simulink model "NoPainNoCrane_Software"  (R2016a)
settings: Solver=ode15s  StartTime=0.0  StopTime=80  RelTol=1e-3
values from neighbouring files (symbols this model uses):
  AngleDX = 0    [RunHWModel.m]    (also in simSetup.m; workspace.mat)
  AngleDY = AngleDX    (= 0)    [RunHWModel.m]    (also in simSetup.m; workspace.mat)
  AngleIX = 0    [RunHWModel.m]    (also in simSetup.m; workspace.mat)
  AngleIY = AngleIX    (= 0)    [RunHWModel.m]    (also in simSetup.m; workspace.mat)
  AnglePX = 2.0    (= 2)    [RunHWModel.m]    (also in simSetup.m; workspace.mat)
  AnglePY = AnglePX    (= 2)    [RunHWModel.m]    (also in simSetup.m; workspace.mat)
  DC1x = 0.1    [RunHWModel.m]    (also in simSetup.m; workspace.mat)
  DC1y = DC1x    (= 0.1)    [RunHWModel.m]    (also in simSetup.m; workspace.mat)
  IC1x = 0.9    [RunHWModel.m]    (also in simSetup.m; workspace.mat)
  IC1y = IC1x    (= 0.9)    [RunHWModel.m]    (also in simSetup.m; workspace.mat)
  m = 0.47    [workspace.mat]
  MR = 1.71    [workspace.mat]
  PC1x = 4.7    [RunHWModel.m]    (also in simSetup.m; workspace.mat)
  PC1y = PC1x    (= 4.7)    [RunHWModel.m]    (also in simSetup.m; workspace.mat)
  TxBreak = 0    [setup.m]    (also in workspace.mat)
  TxCoulomb = 2.5    [setup.m]    (also in workspace.mat)
  TxVisc = 49.1750    (= 49.175)    [setup.m]    (also in workspace.mat)
  TyBreak = 0    [setup.m]    (also in workspace.mat)
  TyCoulomb = 1.8    [setup.m]    (also in workspace.mat)
  TzBreak = 0    [workspace.mat]
  TzCoulomb = 6.1    [workspace.mat]
  waypoints = [waypoints is_target]    [path_planning.m]    (also in workspace.mat = [0 0 9 9 10 6 4 8 19 20 20 0 ... (55 elements, 11x5)])
  xRange = [0 0.52]    [workspace.mat]
  xZero = 0    [setup.m]    (also in workspace.mat)
  yRange = [0 0.62]    [workspace.mat]
  yZero = 0    [setup.m]    (also in workspace.mat)
  zRange = [0.17 0.8]    [workspace.mat]
  zZero = 0.47    [workspace.mat]
undefined symbols (not defined in the file or in its folder): X, Y, Z
undefined symbols (not defined in the file): M, TorqueMultX, TorqueMultY, TorqueMultZ, TxTrans, TyTrans, TyVisc, TzTrans, TzVisc
libraries: sm_lib x146, fl_lib x62, nesl_utility x24, simulink x10, elec_lib x9, sm_double_wishbone_suspension_lib x4, aerolibtransform2 x1
(part 1 of 15)
settings Model: Creator=jsustare  LastModifiedBy=Jukka
settings SolverCC: MaxConsecutiveMinStep=10
settings DataIOCC: SaveFormat=StructureWithTime
settings DebuggingCC: AllowSymbolicDim=off
settings ModelReferenceCC: PropagateSignalLabelsOutOfModel=off
settings GRTTargetCC: GeneratePreprocessorConditionals=Use local settings
settings SimscapeCC: SimscapeLogType=all  SimscapeLogLimitData=off
settings ConfigurationSet: Description=SimMechanics 2G

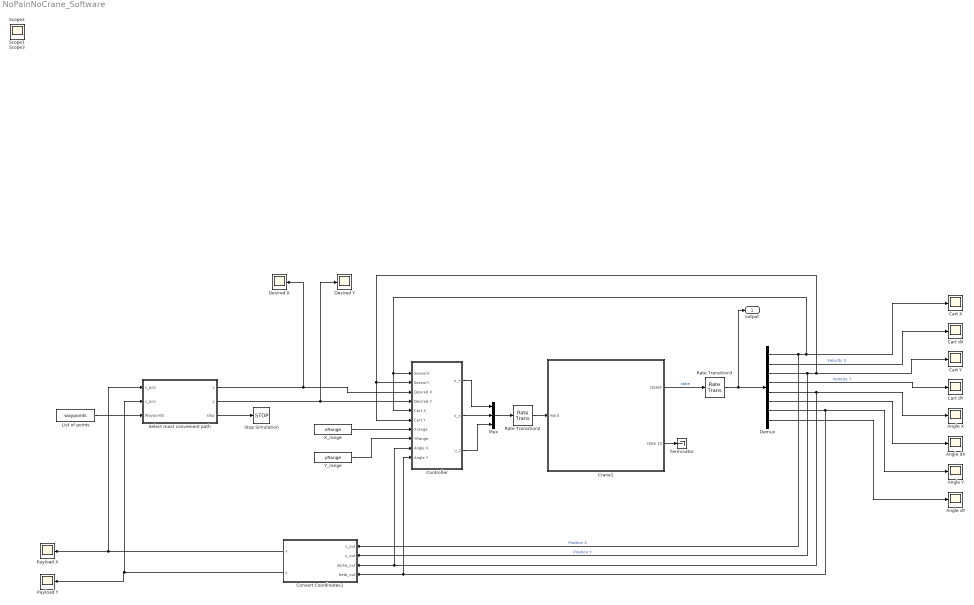
== system NoPainNoCrane_Software ==
  Angle X : Scope
  Angle Y : Scope
  Angle dX : Scope
  Angle dY : Scope
  Cart X : Scope
  Cart Y : Scope
  Cart dX : Scope
  Cart dY : Scope
  Controller : Subsystem
  Convert Coordinates1 : MATLAB Function  TreatAsAtomicUnit=on
  Crane1 : Subsystem  mask{penduMass=m, cartMass=M, MR=MR, xRange=xRange, yRange=yRange, zRange=zRange, xZero=xZero, yZero=yZero, zZero=zZero, TxBreak=TxBreak, TxCoulomb=TxCoulomb, TxVisc=TxVisc, TxTrans=TxTrans, TyBreak=TyBreak, TyCoulomb=TyCoulomb, TyVisc=TyVisc, TyTrans=TyTrans, TzBreak=TzBreak, TzCoulomb=TzCoulomb, TzVisc=TzVisc, TzTrans=TzTrans, Ux=TorqueMultX, Uy=TorqueMultY, Uz=TorqueMultZ}
      mask prompts: penduMass "Pendulum Mass (Kg)"; cartMass "Mass of the cart (Kg)"; MR "Mass of the rail (Kg)"; TxBreak "BreakAwayFriction"; TxCoulomb "Coulomb Friction"; TxVisc "Viscous friction"; TxTrans "Transition coeff"; TyBreak "BreakAwayFriction"; TyCoulomb "Coulomb Friction"; TyVisc "Viscous friction"; TyTrans "Transition coeff"; TzBreak "BreakAwayFriction"; TzCoulomb "Coulomb Friction"; TzVisc "Viscous friction"; TzTrans "Transition coeff"; Ux "Rail motor multiplier (X)"; Uy "Cart motor multiplier (Y)"; Uz "String motor multiplier (Z)"
      mask init:
      | %mass lowSat
      | penduMass=max(penduMass,1e-3);
      | cartMass=max(cartMass,1e-3);
      | MR=max(MR,1e-3);
      | 
      | %zeros saturated
      | xZero=max(xZero,xRange(1));
      | xZero=min(xZero,xRange(2));
      | 
      | yZero=max(yZero,yRange(1));
      | yZero=min(yZero,yRange(2));
      | 
      | zZero=max(zZero,zRange(1));
      | zZero=min(zZero,zRange(2));
      mask DialogControl DescGroupVar Prompt: 3D Crane Simscape model
      mask Display:
